simulink model "yorkToSimu"  (Simulink 7.2)
settings: Solver=ode45  StartTime=0.0  StopTime=10.0  RelTol=1e-3
settings Model: Creator=alesch  LastModifiedBy=alesch

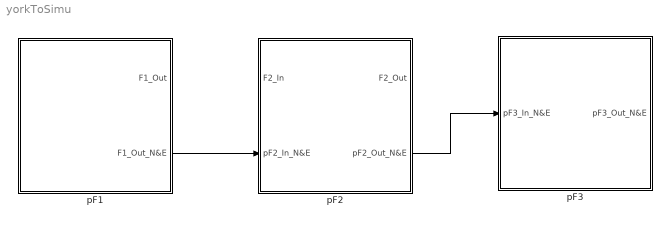
== system yorkToSimu ==
  pF1 : Subsystem
  pF2 : Subsystem
  pF3 : Subsystem
  wires:
  pF1/2(F1_Out_N&E) -> pF2/2(pF2_In_N&E)
  pF2/2(pF2_Out_N&E) -> pF3/1(pF3_In_N&E)

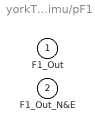
== system yorkToSimu/pF1 ==
  F1_Out : Outport
  F1_Out_N&E : Outport  Port=2

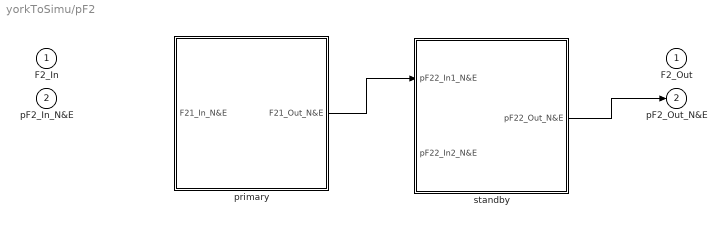
== system yorkToSimu/pF2 ==
  F2_In : Inport
  pF2_In_N&E : Inport  Port=2
  primary : Subsystem
  standby : Subsystem
  F2_Out : Outport
  pF2_Out_N&E : Outport  Port=2
  wires:
  primary/1(F21_Out_N&E) -> standby/1(pF22_In1_N&E)
  standby/1(pF22_Out_N&E) -> pF2_Out_N&E/1

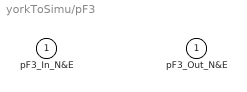
== system yorkToSimu/pF3 ==
  pF3_In_N&E : Inport
  pF3_Out_N&E : Outport

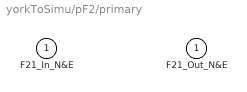
== system yorkToSimu/pF2/primary ==
  F21_In_N&E : Inport
  F21_Out_N&E : Outport

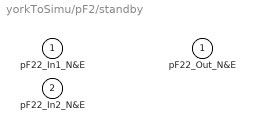
== system yorkToSimu/pF2/standby ==
  pF22_In1_N&E : Inport
  pF22_In2_N&E : Inport  Port=2
  pF22_Out_N&E : Outport
